simulink model "FlightGear_BUS_aerosurface_trim"  (R2017a)
settings: Solver=VariableStepAuto  StartTime=0.0  StopTime=20  FixedStep=0.1  RelTol=1e-5
model workspace (MAT data in the model file):
  handle : class17 (value not decoded)
  handle : class17 (value not decoded)
values from neighbouring files (symbols this model uses):
  a0_s2345 = [0;0;0.05;0.05]    [HW5_4_surfaces.m]    (also in TEST_aerosetup.m; surfaces_setup_test.m)
  A_2345 = c_2345.*b_2345    [HW5_4_surfaces.m]    (also in TEST_aerosetup.m; surfaces_setup_test.m)
  Aileron_left = 0    [HW5_4_surfaces.m]    (also in TEST_aerosetup.m; surfaces_setup_test.m)
  Aileron_right = 0    [HW5_4_surfaces.m]    (also in TEST_aerosetup.m; surfaces_setup_test.m)
  c_2345 = [0.075;0.08;0.1;0.1]    [HW5_4_surfaces.m]    (also in TEST_aerosetup.m; surfaces_setup_test.m)
  CD0_s2345 = [0.01;0.01;0.01;0.01]    [HW5_4_surfaces.m]    (also in TEST_aerosetup.m; surfaces_setup_test.m)
  CDa_s2345 = [1;1;1;1]    [HW5_4_surfaces.m]    (also in TEST_aerosetup.m; surfaces_setup_test.m)
  CL0_2345 = [0;0; 0.05; 0.05]    [HW5_4_surfaces.m]    (also in TEST_aerosetup.m; surfaces_setup_test.m)
  CLa = 2*pi*(r./(2+r))    [HW5_4_surfaces.m]    (also in TEST_aerosetup.m; surfaces_setup_test.m)
  CM0_s2345 = [0;0;-0.05;-0.05]    [HW5_4_surfaces.m]    (also in TEST_aerosetup.m; surfaces_setup_test.m)
  CMa_s2345 = [0; 0; 0; 0]    [HW5_4_surfaces.m]    (also in TEST_aerosetup.m; surfaces_setup_test.m)
  e_s2345 = [0.8;0.8;0.9;0.9]    [HW5_4_surfaces.m]    (also in TEST_aerosetup.m; surfaces_setup_test.m)
  elevator = 0    [HW5_4_surfaces.m]    (also in TEST_aerosetup.m; surfaces_setup_test.m)
  Fext_N = -g_EN * m    [HW5_4_surfaces.m]    (also in TEST_aerosetup.m = [10 10 10]; surfaces_setup_test.m)
  g_EN = [0; 0; 9.81]    [HW5_4_surfaces.m]    (also in TEST_aerosetup.m = [0; 0; 9.8]; surfaces_setup_test.m)
  i_s2345 = [0; 0; 0.05; 0.05;]    [HW5_4_surfaces.m]    (also in TEST_aerosetup.m; surfaces_setup_test.m)
  J_cg = ones(3)    [HW5_4_surfaces.m]    (also in TEST_aerosetup.m)
  J_cgp = ones(3)    [surfaces_setup_test.m]
  M_total = sum(MnG(:,1))/1000    [HW5_4_surfaces.m]    (also in TEST_aerosetup.m; surfaces_setup_test.m = sum(MnG1(:,1))/1000)
  Mext_B = [0; 0; 0]    [HW5_4_surfaces.m]    (also in TEST_aerosetup.m = [1; 1; 1]; surfaces_setup_test.m)
  p_E_BE_ini = p_E_BE_ini_deg .* [deg2rad; deg2rad; 1]    [HW5_4_surfaces.m]    (also in TEST_aerosetup.m; surfaces_setup_test.m)
  r = b_2345./c_2345    [HW5_4_surfaces.m]    (also in TEST_aerosetup.m; surfaces_setup_test.m)
  Rearth = 6371000    [HW5_4_surfaces.m]    (also in TEST_aerosetup.m; surfaces_setup_test.m)
  rudder = 0    [HW5_4_surfaces.m]    (also in TEST_aerosetup.m; surfaces_setup_test.m)
  Theta_ini = Theta_ini_deg * deg2rad    [HW5_4_surfaces.m]    (also in TEST_aerosetup.m; surfaces_setup_test.m)
  v_N_AE = [0;0;0]    [HW5_4_surfaces.m]    (also in TEST_aerosetup.m; surfaces_setup_test.m)
  Vbbe_int = [10; 0; 0]    [HW5_4_surfaces.m]    (also in TEST_aerosetup.m; surfaces_setup_test.m = [5; 0; 0])
  w_B_BE_ini = [1e0; 1e-2; 1e-2]    [HW5_4_surfaces.m]    (also in TEST_aerosetup.m; surfaces_setup_test.m)
  xyz_s = [[-0.76 0 0.16];[-0.76 0 -0.09];[-0.23 0.44 0];[-0.23 -0.44 0];]    [HW5_4_surfaces.m]    (also in TEST_aerosetup.m; surfaces_setup_test.m)
undefined symbols (not defined in the file or in its folder): Earth, WGS84
libraries: dspinverses x6, vrlib x4, simulink x4, aerolibfltsims x3, sharedtransform x2, aerolibtransform2 x2, aerolibutil x1, sharedutil x1
(part 2 of 2)

== matlab function FlightGear_BUS_aerosurface_trim/Subsystem/Rot kine/Euler to Quat 1 ==
  data: att input; H output
function H = fcn(att)
%#codegen
phi=att(1);
theta=att(2);
%psi=theta(3); %not needed for Euler Rotational Kinematics Matrix
H=[1,tan(theta)*sin(phi),tan(theta)*cos(phi); 0,cos(phi),-sin(phi);0,sin(phi)/cos(theta),cos(phi)/cos(theta)];

== matlab function FlightGear_BUS_aerosurface_trim/Subsystem/Rot kine/Euler to Quat 3 ==
  data: att input; Q output
function Q = fcn(att)
phi=att(1);
theta=att(2);
psi=att(3);
q0=cos(phi/2)*cos(theta/2)*cos(psi/2)+sin(phi/2)*sin(theta/2)*sin(psi/2); 
q1=sin(phi/2)*cos(theta/2)*cos(psi/2)-cos(phi/2)*sin(theta/2)*sin(psi/2); 
q2=cos(phi/2)*sin(theta/2)*cos(psi/2)+sin(phi/2)*cos(theta/2)*sin(psi/2); 
q3=cos(phi/2)*cos(theta/2)*sin(psi/2)-sin(phi/2)*sin(theta/2)*cos(psi/2);
Q=[q0;q1;q2;q3];

== matlab function FlightGear_BUS_aerosurface_trim/Subsystem/Rot kine/Quat2Euler 1 ==
  data: Q input; theta output
function theta = fcn(Q)
q0=Q(1);
q1=Q(2);
q2=Q(3);
q3=Q(4);
roll=atan2(2*(q0*q1+q2*q3),q0^2-q1^2-q2^2+q3^2); 
pitch=asin(2*(q0*q2-q1*q3)); 
yaw=atan2(2*(q0*q3+q1*q2),q0^2+q1^2-q2^2-q3^2);
theta=[roll;pitch;yaw];

== matlab function FlightGear_BUS_aerosurface_trim/Subsystem/new tran kine sph/p2Cne/LAT DCM ==
  data: u input; y output
function y = fcn(u)
y = [cos(u) 0 sin(u); 0 1 0; -sin(u) 0 cos(u)];

== matlab function FlightGear_BUS_aerosurface_trim/Subsystem/new tran kine sph/p2Cne/LON DCM ==
  data: u input; y output
function y = fcn(u)

y = [1, 0, 0;0, cos(u), sin(u);0, -sin(u), cos(u)];

== matlab function FlightGear_BUS_aerosurface_trim/Subsystem/new tran kine sph/sph_trans ==
  data: P_BE_E_ini input; X_BE_E_ini output
function X_BE_E_ini = fcn(P_BE_E_ini)
lat=P_BE_E_ini(1);
lon=P_BE_E_ini(2);
alt=P_BE_E_ini(3);
a = 6378000;
e = 8.1819190842622e-2;
N = a ./ sqrt(1 - e^2 .* sin(lat).^2);
x = (N+alt) .* cos(lat) .* cos(lon);
y = (N+alt) .* cos(lat) .* sin(lon);
z = ((1-e^2) .* N + alt) .* sin(lat);
X_BE_E_ini=[(N+alt) .* cos(lat) .* cos(lon); (N+alt) .* cos(lat) .* sin(lon);((1-e^2) .* N + alt) .* sin(lat)];

== matlab function FlightGear_BUS_aerosurface_trim/new tran kine sph/sph_trans ==
  data: P_BE_E_ini input; X_BE_E_ini output
function X_BE_E_ini = fcn(P_BE_E_ini)
lat=P_BE_E_ini(1);
lon=P_BE_E_ini(2);
alt=P_BE_E_ini(3);
a = 6378000;
e = 8.1819190842622e-2;
N = a ./ sqrt(1 - e^2 .* sin(lat).^2);
x = (N+alt) .* cos(lat) .* cos(lon);
y = (N+alt) .* cos(lat) .* sin(lon);
z = ((1-e^2) .* N + alt) .* sin(lat);
X_BE_E_ini=[(N+alt) .* cos(lat) .* cos(lon); (N+alt) .* cos(lat) .* sin(lon);((1-e^2) .* N + alt) .* sin(lat)];
